simulink library "csu_mpl_mass_properties_lander_lib"  (R2015b)
settings: Solver=ode45  StartTime=0.0  StopTime=10.0  RelTol=1e-3
values from neighbouring files (symbols this model uses):
  mpl_cg_dry = [mpl_cgx_location_fillfrac_0 mpl_cgy_location_fillfrac_0 mpl_cgz_location_fillfrac_0]    [csu_mpl_mass_properties_lander_prep.m]
  mpl_gn2_center_tank1 = [  0.4   0.0   0.2]    [csu_mpl_mass_properties_lander_init.m]
  mpl_gn2_center_tank2 = [  0.0   0.4   0.2]    [csu_mpl_mass_properties_lander_init.m]
  mpl_gn2_center_tank3 = [ -0.4   0.0   0.2]    [csu_mpl_mass_properties_lander_init.m]
  mpl_gn2_center_tank4 = [  0.0  -0.4   0.2]    [csu_mpl_mass_properties_lander_init.m]
  mpl_gn2_cg_table = [ mpl_gn2_cg_fillfrac_0;       mpl_gn2_cg_fillfrac_100   ]    [csu_mpl_mass_properties_lander_prep.m]
  mpl_gn2_drain_efficiency_tank1 = 1.0    (= 1)    [csu_mpl_mass_properties_lander_init.m]
  mpl_gn2_drain_efficiency_tank2 = 1.0    (= 1)    [csu_mpl_mass_properties_lander_init.m]
  mpl_gn2_drain_efficiency_tank3 = 1.0    (= 1)    [csu_mpl_mass_properties_lander_init.m]
  mpl_gn2_drain_efficiency_tank4 = 1.0    (= 1)    [csu_mpl_mass_properties_lander_init.m]
  mpl_gn2_inertia_table_tank1 = [ buildInertiaVector(mpl_gn2_inertia_fillfrac_0_tank1);  buildInertiaVector(mpl_gn2_inertia_fillfrac_100_tank1) ]    [csu_mpl_mass_properties_lander_prep.m]
  mpl_gn2_inertia_table_tank2 = [ buildInertiaVector(mpl_gn2_inertia_fillfrac_0_tank2);  buildInertiaVector(mpl_gn2_inertia_fillfrac_100_tank2) ]    [csu_mpl_mass_properties_lander_prep.m]
  mpl_gn2_inertia_table_tank3 = [ buildInertiaVector(mpl_gn2_inertia_fillfrac_0_tank3);  buildInertiaVector(mpl_gn2_inertia_fillfrac_100_tank3) ]    [csu_mpl_mass_properties_lander_prep.m]
  mpl_gn2_inertia_table_tank4 = [ buildInertiaVector(mpl_gn2_inertia_fillfrac_0_tank4);  buildInertiaVector(mpl_gn2_inertia_fillfrac_100_tank4) ]    [csu_mpl_mass_properties_lander_prep.m]
  mpl_gn2_mass_initial_tank1 = 0.5    [csu_mpl_mass_properties_lander_init.m]    (also in csu_mpl_mass_properties_lander_prep.m = mpl_gn2_mass_initial/4)
  mpl_gn2_mass_initial_tank2 = 0.5    [csu_mpl_mass_properties_lander_init.m]    (also in csu_mpl_mass_properties_lander_prep.m = mpl_gn2_mass_initial/4)
  mpl_gn2_mass_initial_tank3 = 0.5    [csu_mpl_mass_properties_lander_init.m]    (also in csu_mpl_mass_properties_lander_prep.m = mpl_gn2_mass_initial/4)
  mpl_gn2_mass_initial_tank4 = 0.5    [csu_mpl_mass_properties_lander_init.m]    (also in csu_mpl_mass_properties_lander_prep.m = mpl_gn2_mass_initial/4)
  mpl_gn2_mass_table = [ mpl_gn2_mass_fillfrac_0;     mpl_gn2_mass_fillfrac_100 ]    [csu_mpl_mass_properties_lander_prep.m]
  mpl_htp_cg_table = [ mpl_htp_cg_fillfrac_0;     mpl_htp_cg_fillfrac_100   ]    [csu_mpl_mass_properties_lander_prep.m]
  mpl_htp_inertia_table = [ buildInertiaVector(mpl_htp_inertia_fillfrac_0);  buildInertiaVector(mpl_htp_inertia_fillfrac_100) ]    [csu_mpl_mass_properties_lander_prep.m]
  mpl_htp_mass_initial = 317.68    [csu_mpl_mass_properties_lander_init.m]
  mpl_htp_mass_table = [ mpl_htp_mass_fillfrac_0;   mpl_htp_mass_fillfrac_100 ]    [csu_mpl_mass_properties_lander_prep.m]
  mpl_htp_tank_center = [  0.0  0.0  0.4]    [csu_mpl_mass_properties_lander_init.m]
  mpl_inertia_dry = buildInertiaMatrix(mpl_inertia_fillfrac_0([1 2 3 4 6 5]))    [csu_mpl_mass_properties_lander_prep.m]
  mpl_mass_dry = 123.9    [csu_mpl_mass_properties_lander_init_scn_4.m]    (also in csu_mpl_mass_properties_lander_prep.m = mpl_mass_fillfrac_0)
  mpl_rp1_cg_table = [ mpl_rp1_cg_fillfrac_0;     mpl_rp1_cg_fillfrac_100   ]    [csu_mpl_mass_properties_lander_prep.m]
  mpl_rp1_inertia_table = [ buildInertiaVector(mpl_rp1_inertia_fillfrac_0);  buildInertiaVector(mpl_rp1_inertia_fillfrac_100) ]    [csu_mpl_mass_properties_lander_prep.m]
  mpl_rp1_mass_initial = 79.42    [csu_mpl_mass_properties_lander_init.m]
  mpl_rp1_mass_table = [ mpl_rp1_mass_fillfrac_0;   mpl_rp1_mass_fillfrac_100 ]    [csu_mpl_mass_properties_lander_prep.m]
  mpl_rp1_tank_center = [  0.0  0.0  0.1]    [csu_mpl_mass_properties_lander_init.m]
libraries: util_mass_prop_lib x14, simulink x4, util_common_lib x2, util_info_lib x1, util_quat_lib x1
settings Model: Creator=Mark Agbayani  LastModifiedBy=jimkaidy
settings DataIOCC: SaveFormat=Array
settings DebuggingCC: SolverPrmCheckMsg=warning
settings HardwareCC: ProdBitPerPointer=32  ProdLargestAtomicFloat=None  ProdIntDivRoundTo=Undefined  ProdEndianess=Unspecified  ProdWordSize=32  ProdHWDeviceType=32-bit Generic
settings GRTTargetCC: GeneratePreprocessorConditionals=Disable all
settings ConfigComp: CovModelRefEnable=Off  CovSFcnEnable=off

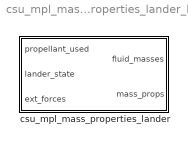
== system csu_mpl_mass_properties_lander_lib ==
  csu_mpl_mass_properties_lander : Subsystem

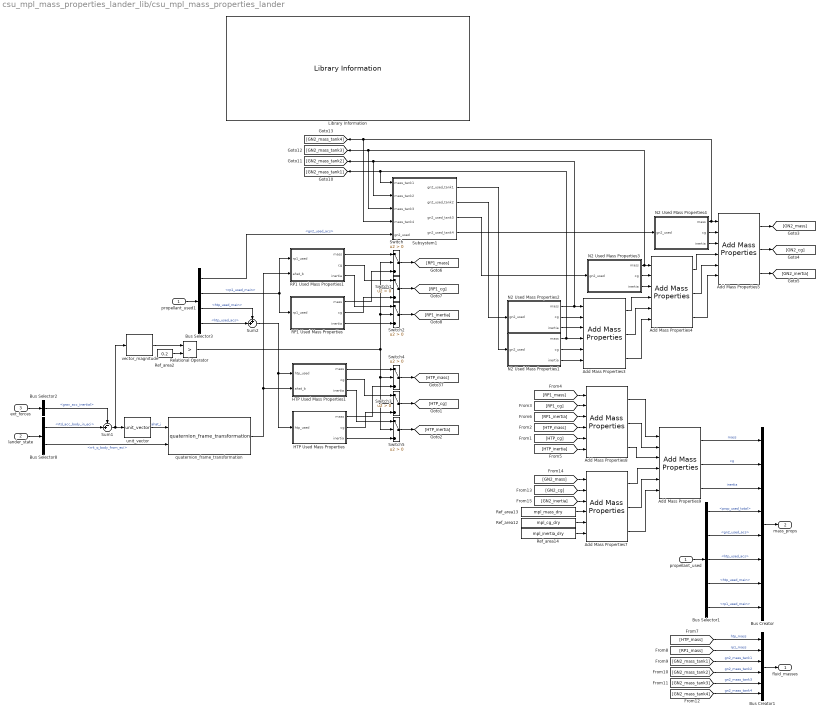
== system csu_mpl_mass_properties_lander_lib/csu_mpl_mass_properties_lander ==
  propellant_used : Inport
  lander_state : Inport  Port=2
  ext_forces : Inport  Port=3
  Add Mass Properties{3..5,7..9} (6 alike) : util_mass_prop_lib/Add Mass Properties  SystemSampleTime=-1
  Bus Creator : BusCreator  Inputs=8  OutDataTypeStr=Bus: mass_props_msg_t
  Bus Creator1 : BusCreator  Inputs=6
  Bus Selector1 : BusSelector  OutputSignals=prop_used_total,gn2_used_acs,htp_used_acs,htp_used_main,rp1_used_main
  Bus Selector2 : BusSelector  OutputSignals=grav_acc_inertial
  Bus Selector3 : BusSelector  OutputSignals=gn2_used_acs,rp1_used_main,htp_used_main,htp_used_acs
  Bus Selector8 : BusSelector  OutputSignals=rtd_acc_body_in_eci,rrk_q_body_from_eci
  HTP Used Mass Properties : Subsystem
  HTP Used Mass Properties1 : Subsystem
  Library Information : util_info_lib/Library Information  owner='NONE'
  N2 Used Mass Properties1 : Subsystem
  N2 Used Mass Properties2 : Subsystem
  N2 Used Mass Properties3 : Subsystem
  N2 Used Mass Properties4 : Subsystem
  RP1 Used Mass Properties : Subsystem
  RP1 Used Mass Properties1 : Subsystem
  Ref_area12 : Constant  Value=mpl_cg_dry
  Ref_area13 : Constant  Value=mpl_mass_dry
  Ref_area14 : Constant  Value=mpl_inertia_dry
  Ref_area2 : Constant  Value=0.2
  Relational Operator : RelationalOperator  Operator=>  OutDataTypeStr=boolean
  Subsystem1 : Subsystem
  Sum1 : Sum  Inputs=-+|
  Sum2 : Sum  Inputs=++|
  Switch{,1..5} (6 alike) : Switch  Criteria=u2 > Threshold
  propellant_used1 : InportShadow
  quaternion_frame_transformation : util_quat_lib/quaternion_frame_transformation  SystemSampleTime=-1
  unit_vector : util_common_lib/unit_vector  SystemSampleTime=-1
  vector_magnitude : util_common_lib/vector_magnitude  SystemSampleTime=-1
  fluid_masses : Outport
  mass_props : Outport  Port=2
  wires:
  Bus Selector8/1 -> Sum1/2  "<rtd_acc_body_in_eci>"
  Bus Selector2/1 -> Sum1/1  "<grav_acc_inertial>"
  ext_forces/1 -> Bus Selector2/1
  Sum1/1 -> unit_vector/1, vector_magnitude/1
  Relational Operator/1 -> Switch2/2, Switch1/2, Switch/2, Switch4/2, Switch5/2, Switch3/2
  Switch3/1 -> [HTP_cg]
  Switch5/1 -> [HTP_inertia]
  Switch4/1 -> [HTP_mass]
  HTP Used Mass Properties/3(inertia) -> Switch5/3
  HTP Used Mass Properties1/3(inertia) -> Switch5/1
  HTP Used Mass Properties/2(cg) -> Switch3/3
  HTP Used Mass Properties1/2(cg) -> Switch3/1
  HTP Used Mass Properties/1(mass) -> Switch4/3
  HTP Used Mass Properties1/1(mass) -> Switch4/1
  RP1 Used Mass Properties/3(inertia) -> Switch2/3
  RP1 Used Mass Properties1/3(inertia) -> Switch2/1
  RP1 Used Mass Properties/2(cg) -> Switch1/3
  RP1 Used Mass Properties1/2(cg) -> Switch1/1
  RP1 Used Mass Properties/1(mass) -> Switch/3
  RP1 Used Mass Properties1/1(mass) -> Switch/1
  Switch2/1 -> [RP1_inertia]
  Switch1/1 -> [RP1_cg]
  Switch/1 -> [RP1_mass]
  Ref_area2/1 -> Relational Operator/2
  vector_magnitude/1 -> Relational Operator/1
  quaternion_frame_transformation/1 -> RP1 Used Mass Properties1/2(ahat_b), HTP Used Mass Properties1/2(ahat_b)
  Bus Selector3/1 -> Subsystem1/5(gn2_used)  "<gn2_used_acs>"
  Bus Selector1/5 -> Bus Creator/8  "<rp1_used_main>"
  Bus Selector1/2 -> Bus Creator/5  "<gn2_used_acs>"
  [GN2_inertia] -> Add Mass Properties7/3
  [GN2_cg] -> Add Mass Properties7/2
  [GN2_mass] -> Add Mass Properties7/1
  Add Mass Properties7/3 -> Add Mass Properties9/6
  Add Mass Properties7/2 -> Add Mass Properties9/5
  Add Mass Properties7/1 -> Add Mass Properties9/4
  Sum2/1 -> HTP Used Mass Properties1/1(htp_used), HTP Used Mass Properties/1(htp_used)
  Bus Selector3/4 -> Sum2/2  "<htp_used_acs>"
  Bus Selector3/2 -> RP1 Used Mass Properties/1(rp1_used), RP1 Used Mass Properties1/1(rp1_used)  "<rp1_used_main>"
  unit_vector/1 -> quaternion_frame_transformation/1  "ahat_i"
  Bus Selector8/2 -> quaternion_frame_transformation/2  "<rrk_q_body_from_eci>"
  lander_state/1 -> Bus Selector8/1
  [GN2_mass_tank4] -> Bus Creator1/6  "gn2_mass_tank4"
  [GN2_mass_tank3] -> Bus Creator1/5  "gn2_mass_tank3"
  [GN2_mass_tank2] -> Bus Creator1/4  "gn2_mass_tank2"
  [GN2_mass_tank1] -> Bus Creator1/3  "gn2_mass_tank1"
  [HTP_mass] -> Bus Creator1/1  "htp_mass"
  Bus Creator1/1 -> fluid_masses/1
  Subsystem1/1(gn2_used_tank1) -> N2 Used Mass Properties1/1(gn2_used)
  Subsystem1/2(gn2_used_tank2) -> N2 Used Mass Properties2/1(gn2_used)
  Subsystem1/3(gn2_used_tank3) -> N2 Used Mass Properties3/1(gn2_used)
  Subsystem1/4(gn2_used_tank4) -> N2 Used Mass Properties4/1(gn2_used)
  Ref_area12/1 -> Add Mass Properties7/5
  N2 Used Mass Properties4/1(mass) -> Add Mass Properties5/1, Subsystem1/4(mass_tank4), [GN2_mass_tank4]
  N2 Used Mass Properties3/1(mass) -> Add Mass Properties4/1, Subsystem1/3(mass_tank3), [GN2_mass_tank3]
  N2 Used Mass Properties2/1(mass) -> Add Mass Properties3/1, Subsystem1/2(mass_tank2), [GN2_mass_tank2]
  N2 Used Mass Properties1/1(mass) -> Add Mass Properties3/4, [GN2_mass_tank1], Subsystem1/1(mass_tank1)
  Ref_area13/1 -> Add Mass Properties7/4
  Ref_area14/1 -> Add Mass Properties7/6
  N2 Used Mass Properties1/2(cg) -> Add Mass Properties3/5
  N2 Used Mass Properties1/3(inertia) -> Add Mass Properties3/6
  N2 Used Mass Properties2/3(inertia) -> Add Mass Properties3/3
  N2 Used Mass Properties2/2(cg) -> Add Mass Properties3/2
  Add Mass Properties3/1 -> Add Mass Properties4/4
  Add Mass Properties3/2 -> Add Mass Properties4/5
  Add Mass Properties3/3 -> Add Mass Properties4/6
  N2 Used Mass Properties3/3(inertia) -> Add Mass Properties4/3
  N2 Used Mass Properties3/2(cg) -> Add Mass Properties4/2
  N2 Used Mass Properties4/2(cg) -> Add Mass Properties5/2
  N2 Used Mass Properties4/3(inertia) -> Add Mass Properties5/3
  Add Mass Properties4/1 -> Add Mass Properties5/4
  Add Mass Properties4/2 -> Add Mass Properties5/5
  Add Mass Properties4/3 -> Add Mass Properties5/6
  Add Mass Properties5/1 -> [GN2_mass]
  Add Mass Properties5/2 -> [GN2_cg]
  Add Mass Properties5/3 -> [GN2_inertia]
  [HTP_inertia] -> Add Mass Properties8/6
  [HTP_cg] -> Add Mass Properties8/5
  [HTP_mass] -> Add Mass Properties8/4
  [RP1_inertia] -> Add Mass Properties8/3
  [RP1_cg] -> Add Mass Properties8/2
  [RP1_mass] -> Add Mass Properties8/1
  Add Mass Properties8/3 -> Add Mass Properties9/3
  Add Mass Properties8/2 -> Add Mass Properties9/2
  Add Mass Properties8/1 -> Add Mass Properties9/1
  Bus Selector3/3 -> Sum2/1  "<htp_used_main>"
  Bus Creator/1 -> mass_props/1
  Bus Selector1/1 -> Bus Creator/4  "<prop_used_total>"
  Bus Selector1/3 -> Bus Creator/6  "<htp_used_acs>"
  Bus Selector1/4 -> Bus Creator/7  "<htp_used_main>"
  Add Mass Properties9/1 -> Bus Creator/1  "mass"
  Add Mass Properties9/2 -> Bus Creator/2  "cg"
  Add Mass Properties9/3 -> Bus Creator/3  "inertia"
  propellant_used/1 -> Bus Selector1/1
  propellant_used1/1 -> Bus Selector3/1
  [RP1_mass] -> Bus Creator1/2  "rp1_mass"

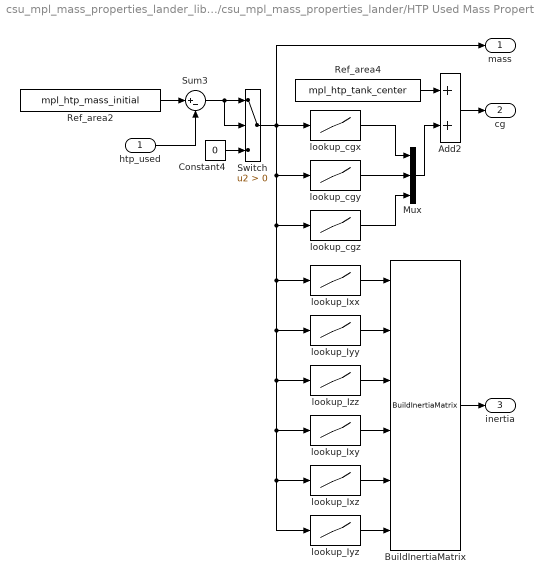
== system csu_mpl_mass_properties_lander_lib/csu_mpl_mass_properties_lander/HTP Used Mass Properties ==
  htp_used : Inport
  Add2 : Sum
  BuildInertiaMatrix : util_mass_prop_lib/BuildInertiaMatrix  SystemSampleTime=-1
  Constant4 : Constant  Value=0
  Mux : Mux  Inputs=3
  Ref_area2 : Constant  Value=mpl_htp_mass_initial
  Ref_area4 : Constant  Value=mpl_htp_tank_center
  Sum3 : Sum  Inputs=|+-
  Switch : Switch  Criteria=u2 > Threshold  SaturateOnIntegerOverflow=on
  lookup_Ixx : Lookup  InputValues=mpl_htp_mass_table  Table=mpl_htp_inertia_table(:,1)
  lookup_Ixy : Lookup  InputValues=mpl_htp_mass_table  Table=mpl_htp_inertia_table(:,4)
  lookup_Ixz : Lookup  InputValues=mpl_htp_mass_table  Table=mpl_htp_inertia_table(:,5)
  lookup_Iyy : Lookup  InputValues=mpl_htp_mass_table  Table=mpl_htp_inertia_table(:,2)
  lookup_Iyz : Lookup  InputValues=mpl_htp_mass_table  Table=mpl_htp_inertia_table(:,6)
  lookup_Izz : Lookup  InputValues=mpl_htp_mass_table  Table=mpl_htp_inertia_table(:,3)
  lookup_cgx : Lookup  InputValues=mpl_htp_mass_table  Table=mpl_htp_cg_table(:,1)
  lookup_cgy : Lookup  InputValues=mpl_htp_mass_table  Table=mpl_htp_cg_table(:,2)
  lookup_cgz : Lookup  InputValues=mpl_htp_mass_table  Table=mpl_htp_cg_table(:,3)
  mass : Outport
  cg : Outport  Port=2
  inertia : Outport  Port=3
  wires:
  Mux/1 -> Add2/2
  lookup_cgy/1 -> Mux/2
  lookup_cgz/1 -> Mux/3
  Ref_area4/1 -> Add2/1
  lookup_Ixx/1 -> BuildInertiaMatrix/1
  lookup_Iyy/1 -> BuildInertiaMatrix/2
  lookup_Izz/1 -> BuildInertiaMatrix/3
  lookup_Ixy/1 -> BuildInertiaMatrix/4
  lookup_Ixz/1 -> BuildInertiaMatrix/5
  lookup_Iyz/1 -> BuildInertiaMatrix/6
  BuildInertiaMatrix/1 -> inertia/1
  lookup_cgx/1 -> Mux/1
  Ref_area2/1 -> Sum3/1
  htp_used/1 -> Sum3/2
  Add2/1 -> cg/1
  Switch/1 -> mass/1, lookup_cgx/1, lookup_cgy/1, lookup_cgz/1, lookup_Ixx/1, lookup_Iyy/1, lookup_Izz/1, lookup_Ixy/1, lookup_Ixz/1, lookup_Iyz/1
  Sum3/1 -> Switch/2, Switch/1
  Constant4/1 -> Switch/3

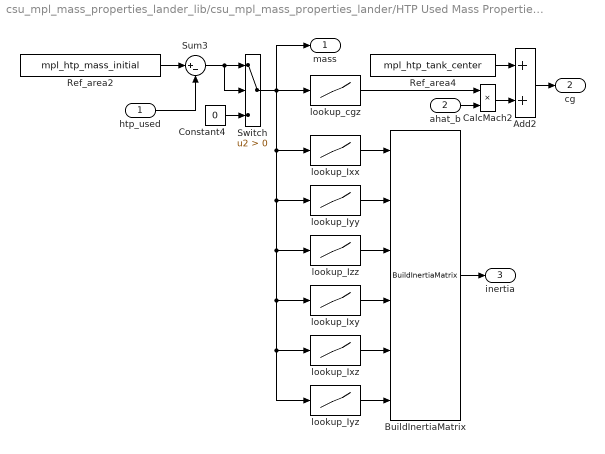
== system csu_mpl_mass_properties_lander_lib/csu_mpl_mass_properties_lander/HTP Used Mass Properties1 ==
  htp_used : Inport
  ahat_b : Inport  Port=2
  Add2 : Sum
  BuildInertiaMatrix : util_mass_prop_lib/BuildInertiaMatrix  SystemSampleTime=-1
  CalcMach2 : Product  SaturateOnIntegerOverflow=on  OutDataTypeStr=Inherit: Same as first input
  Constant4 : Constant  Value=0
  Ref_area2 : Constant  Value=mpl_htp_mass_initial
  Ref_area4 : Constant  Value=mpl_htp_tank_center
  Sum3 : Sum  Inputs=|+-
  Switch : Switch  Criteria=u2 > Threshold  SaturateOnIntegerOverflow=on
  lookup_Ixx : Lookup  InputValues=mpl_htp_mass_table  Table=mpl_htp_inertia_table(:,1)
  lookup_Ixy : Lookup  InputValues=mpl_htp_mass_table  Table=mpl_htp_inertia_table(:,4)
  lookup_Ixz : Lookup  InputValues=mpl_htp_mass_table  Table=mpl_htp_inertia_table(:,5)
  lookup_Iyy : Lookup  InputValues=mpl_htp_mass_table  Table=mpl_htp_inertia_table(:,2)
  lookup_Iyz : Lookup  InputValues=mpl_htp_mass_table  Table=mpl_htp_inertia_table(:,6)
  lookup_Izz : Lookup  InputValues=mpl_htp_mass_table  Table=mpl_htp_inertia_table(:,3)
  lookup_cgz : Lookup  InputValues=mpl_htp_mass_table  Table=mpl_htp_cg_table(:,3)
  mass : Outport
  cg : Outport  Port=2
  inertia : Outport  Port=3
  wires:
  Add2/1 -> cg/1
  htp_used/1 -> Sum3/2
  Ref_area2/1 -> Sum3/1
  BuildInertiaMatrix/1 -> inertia/1
  lookup_Iyz/1 -> BuildInertiaMatrix/6
  lookup_Ixz/1 -> BuildInertiaMatrix/5
  lookup_Ixy/1 -> BuildInertiaMatrix/4
  lookup_Izz/1 -> BuildInertiaMatrix/3
  lookup_Iyy/1 -> BuildInertiaMatrix/2
  lookup_Ixx/1 -> BuildInertiaMatrix/1
  Ref_area4/1 -> Add2/1
  CalcMach2/1 -> Add2/2
  Switch/1 -> mass/1, lookup_Iyz/1, lookup_Ixz/1, lookup_Ixy/1, lookup_Izz/1, lookup_Iyy/1, lookup_Ixx/1, lookup_cgz/1
  Sum3/1 -> Switch/2, Switch/1
  Constant4/1 -> Switch/3
  lookup_cgz/1 -> CalcMach2/1
  ahat_b/1 -> CalcMach2/2

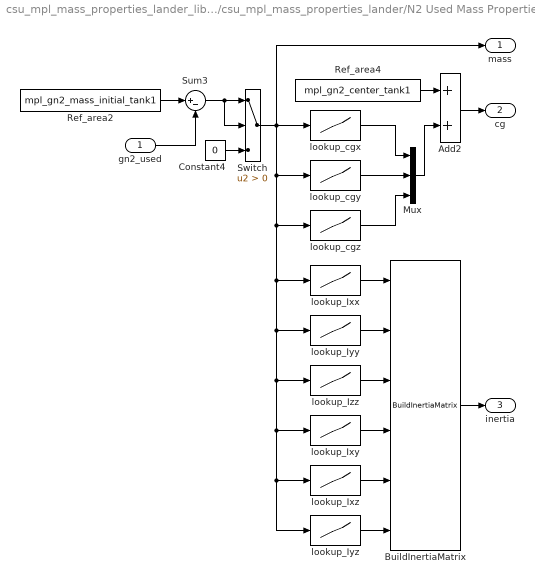
== system csu_mpl_mass_properties_lander_lib/csu_mpl_mass_properties_lander/N2 Used Mass Properties1 ==
  gn2_used : Inport
  Add2 : Sum
  BuildInertiaMatrix : util_mass_prop_lib/BuildInertiaMatrix  SystemSampleTime=-1
  Constant4 : Constant  Value=0
  Mux : Mux  Inputs=3
  Ref_area2 : Constant  Value=mpl_gn2_mass_initial_tank1
  Ref_area4 : Constant  Value=mpl_gn2_center_tank1
  Sum3 : Sum  Inputs=|+-
  Switch : Switch  Criteria=u2 > Threshold  SaturateOnIntegerOverflow=on
  lookup_Ixx : Lookup  InputValues=mpl_gn2_mass_table  Table=mpl_gn2_inertia_table_tank1(:,1)
  lookup_Ixy : Lookup  InputValues=mpl_gn2_mass_table  Table=mpl_gn2_inertia_table_tank1(:,4)
  lookup_Ixz : Lookup  InputValues=mpl_gn2_mass_table  Table=mpl_gn2_inertia_table_tank1(:,5)
  lookup_Iyy : Lookup  InputValues=mpl_gn2_mass_table  Table=mpl_gn2_inertia_table_tank1(:,2)
  lookup_Iyz : Lookup  InputValues=mpl_gn2_mass_table  Table=mpl_gn2_inertia_table_tank1(:,6)
  lookup_Izz : Lookup  InputValues=mpl_gn2_mass_table  Table=mpl_gn2_inertia_table_tank1(:,3)
  lookup_cgx : Lookup  InputValues=mpl_gn2_mass_table  Table=mpl_gn2_cg_table(:,1)
  lookup_cgy : Lookup  InputValues=mpl_gn2_mass_table  Table=mpl_gn2_cg_table(:,2)
  lookup_cgz : Lookup  InputValues=mpl_gn2_mass_table  Table=mpl_gn2_cg_table(:,3)
  mass : Outport
  cg : Outport  Port=2
  inertia : Outport  Port=3
  wires:
  Constant4/1 -> Switch/3
  Sum3/1 -> Switch/1, Switch/2
  Switch/1 -> lookup_Iyz/1, lookup_Ixz/1, lookup_Ixy/1, lookup_Izz/1, lookup_Iyy/1, lookup_Ixx/1, lookup_cgz/1, lookup_cgy/1, lookup_cgx/1, mass/1
  Add2/1 -> cg/1
  gn2_used/1 -> Sum3/2
  Ref_area2/1 -> Sum3/1
  lookup_cgx/1 -> Mux/1
  BuildInertiaMatrix/1 -> inertia/1
  lookup_Iyz/1 -> BuildInertiaMatrix/6
  lookup_Ixz/1 -> BuildInertiaMatrix/5
  lookup_Ixy/1 -> BuildInertiaMatrix/4
  lookup_Izz/1 -> BuildInertiaMatrix/3
  lookup_Iyy/1 -> BuildInertiaMatrix/2
  lookup_Ixx/1 -> BuildInertiaMatrix/1
  Ref_area4/1 -> Add2/1
  lookup_cgz/1 -> Mux/3
  lookup_cgy/1 -> Mux/2
  Mux/1 -> Add2/2

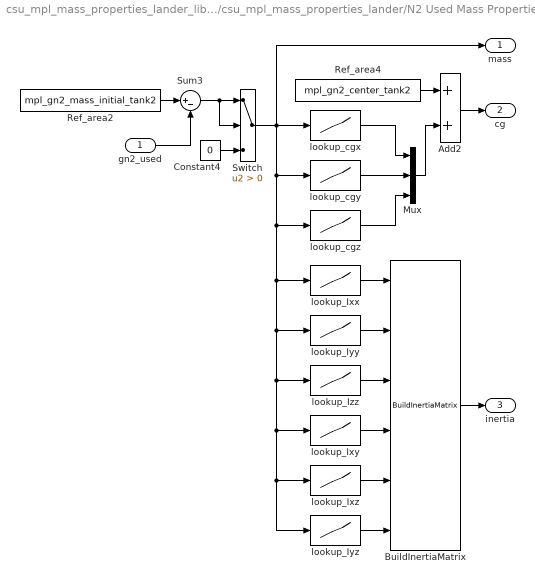
== system csu_mpl_mass_properties_lander_lib/csu_mpl_mass_properties_lander/N2 Used Mass Properties2 ==
  gn2_used : Inport
  Add2 : Sum
  BuildInertiaMatrix : util_mass_prop_lib/BuildInertiaMatrix  SystemSampleTime=-1
  Constant4 : Constant  Value=0
  Mux : Mux  Inputs=3
  Ref_area2 : Constant  Value=mpl_gn2_mass_initial_tank2
  Ref_area4 : Constant  Value=mpl_gn2_center_tank2
  Sum3 : Sum  Inputs=|+-
  Switch : Switch  Criteria=u2 > Threshold  SaturateOnIntegerOverflow=on
  lookup_Ixx : Lookup  InputValues=mpl_gn2_mass_table  Table=mpl_gn2_inertia_table_tank2(:,1)
  lookup_Ixy : Lookup  InputValues=mpl_gn2_mass_table  Table=mpl_gn2_inertia_table_tank2(:,4)
  lookup_Ixz : Lookup  InputValues=mpl_gn2_mass_table  Table=mpl_gn2_inertia_table_tank2(:,5)
  lookup_Iyy : Lookup  InputValues=mpl_gn2_mass_table  Table=mpl_gn2_inertia_table_tank2(:,2)
  lookup_Iyz : Lookup  InputValues=mpl_gn2_mass_table  Table=mpl_gn2_inertia_table_tank2(:,6)
  lookup_Izz : Lookup  InputValues=mpl_gn2_mass_table  Table=mpl_gn2_inertia_table_tank2(:,3)
  lookup_cgx : Lookup  InputValues=mpl_gn2_mass_table  Table=mpl_gn2_cg_table(:,1)
  lookup_cgy : Lookup  InputValues=mpl_gn2_mass_table  Table=mpl_gn2_cg_table(:,2)
  lookup_cgz : Lookup  InputValues=mpl_gn2_mass_table  Table=mpl_gn2_cg_table(:,3)
  mass : Outport
  cg : Outport  Port=2
  inertia : Outport  Port=3
  wires:
  Constant4/1 -> Switch/3
  Sum3/1 -> Switch/1, Switch/2
  Switch/1 -> lookup_cgx/1, lookup_cgy/1, lookup_cgz/1, lookup_Ixx/1, lookup_Iyy/1, lookup_Izz/1, lookup_Ixy/1, lookup_Ixz/1, lookup_Iyz/1, mass/1
  Mux/1 -> Add2/2
  lookup_cgy/1 -> Mux/2
  lookup_cgz/1 -> Mux/3
  Ref_area4/1 -> Add2/1
  lookup_Ixx/1 -> BuildInertiaMatrix/1
  lookup_Iyy/1 -> BuildInertiaMatrix/2
  lookup_Izz/1 -> BuildInertiaMatrix/3
  lookup_Ixy/1 -> BuildInertiaMatrix/4
  lookup_Ixz/1 -> BuildInertiaMatrix/5
  lookup_Iyz/1 -> BuildInertiaMatrix/6
  BuildInertiaMatrix/1 -> inertia/1
  lookup_cgx/1 -> Mux/1
  Ref_area2/1 -> Sum3/1
  gn2_used/1 -> Sum3/2
  Add2/1 -> cg/1

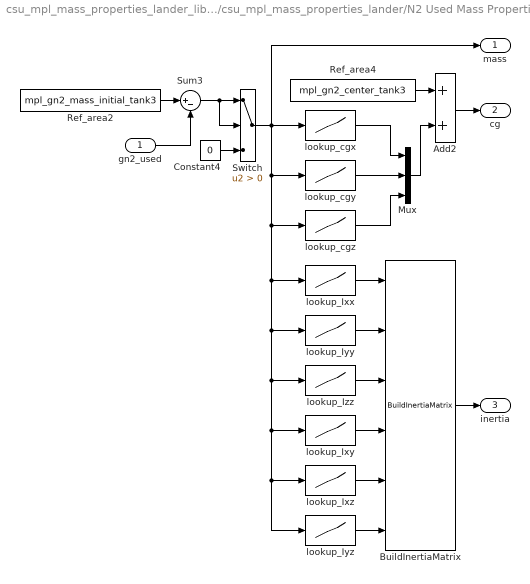
== system csu_mpl_mass_properties_lander_lib/csu_mpl_mass_properties_lander/N2 Used Mass Properties3 ==
  gn2_used : Inport
  Add2 : Sum
  BuildInertiaMatrix : util_mass_prop_lib/BuildInertiaMatrix  SystemSampleTime=-1
  Constant4 : Constant  Value=0
  Mux : Mux  Inputs=3
  Ref_area2 : Constant  Value=mpl_gn2_mass_initial_tank3
  Ref_area4 : Constant  Value=mpl_gn2_center_tank3
  Sum3 : Sum  Inputs=|+-
  Switch : Switch  Criteria=u2 > Threshold  SaturateOnIntegerOverflow=on
  lookup_Ixx : Lookup  InputValues=mpl_gn2_mass_table  Table=mpl_gn2_inertia_table_tank3(:,1)
  lookup_Ixy : Lookup  InputValues=mpl_gn2_mass_table  Table=mpl_gn2_inertia_table_tank3(:,4)
  lookup_Ixz : Lookup  InputValues=mpl_gn2_mass_table  Table=mpl_gn2_inertia_table_tank3(:,5)
  lookup_Iyy : Lookup  InputValues=mpl_gn2_mass_table  Table=mpl_gn2_inertia_table_tank3(:,2)
  lookup_Iyz : Lookup  InputValues=mpl_gn2_mass_table  Table=mpl_gn2_inertia_table_tank3(:,6)
  lookup_Izz : Lookup  InputValues=mpl_gn2_mass_table  Table=mpl_gn2_inertia_table_tank3(:,3)
  lookup_cgx : Lookup  InputValues=mpl_gn2_mass_table  Table=mpl_gn2_cg_table(:,1)
  lookup_cgy : Lookup  InputValues=mpl_gn2_mass_table  Table=mpl_gn2_cg_table(:,2)
  lookup_cgz : Lookup  InputValues=mpl_gn2_mass_table  Table=mpl_gn2_cg_table(:,3)
  mass : Outport
  cg : Outport  Port=2
  inertia : Outport  Port=3
  wires:
  Constant4/1 -> Switch/3
  Sum3/1 -> Switch/1, Switch/2
  Switch/1 -> lookup_cgx/1, mass/1, lookup_Iyz/1, lookup_Ixz/1, lookup_Ixy/1, lookup_Izz/1, lookup_Iyy/1, lookup_Ixx/1, lookup_cgz/1, lookup_cgy/1
  Add2/1 -> cg/1
  gn2_used/1 -> Sum3/2
  Ref_area2/1 -> Sum3/1
  lookup_cgx/1 -> Mux/1
  BuildInertiaMatrix/1 -> inertia/1
  lookup_Iyz/1 -> BuildInertiaMatrix/6
  lookup_Ixz/1 -> BuildInertiaMatrix/5
  lookup_Ixy/1 -> BuildInertiaMatrix/4
  lookup_Izz/1 -> BuildInertiaMatrix/3
  lookup_Iyy/1 -> BuildInertiaMatrix/2
  lookup_Ixx/1 -> BuildInertiaMatrix/1
  Ref_area4/1 -> Add2/1
  lookup_cgz/1 -> Mux/3
  lookup_cgy/1 -> Mux/2
  Mux/1 -> Add2/2

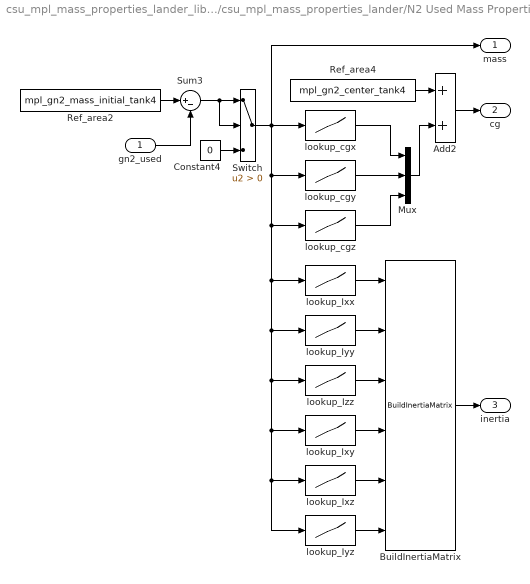
== system csu_mpl_mass_properties_lander_lib/csu_mpl_mass_properties_lander/N2 Used Mass Properties4 ==
  gn2_used : Inport
  Add2 : Sum
  BuildInertiaMatrix : util_mass_prop_lib/BuildInertiaMatrix  SystemSampleTime=-1
  Constant4 : Constant  Value=0
  Mux : Mux  Inputs=3
  Ref_area2 : Constant  Value=mpl_gn2_mass_initial_tank4
  Ref_area4 : Constant  Value=mpl_gn2_center_tank4
  Sum3 : Sum  Inputs=|+-
  Switch : Switch  Criteria=u2 > Threshold  SaturateOnIntegerOverflow=on
  lookup_Ixx : Lookup  InputValues=mpl_gn2_mass_table  Table=mpl_gn2_inertia_table_tank4(:,1)
  lookup_Ixy : Lookup  InputValues=mpl_gn2_mass_table  Table=mpl_gn2_inertia_table_tank4(:,4)
  lookup_Ixz : Lookup  InputValues=mpl_gn2_mass_table  Table=mpl_gn2_inertia_table_tank4(:,5)
  lookup_Iyy : Lookup  InputValues=mpl_gn2_mass_table  Table=mpl_gn2_inertia_table_tank4(:,2)
  lookup_Iyz : Lookup  InputValues=mpl_gn2_mass_table  Table=mpl_gn2_inertia_table_tank4(:,6)
  lookup_Izz : Lookup  InputValues=mpl_gn2_mass_table  Table=mpl_gn2_inertia_table_tank4(:,3)
  lookup_cgx : Lookup  InputValues=mpl_gn2_mass_table  Table=mpl_gn2_cg_table(:,1)
  lookup_cgy : Lookup  InputValues=mpl_gn2_mass_table  Table=mpl_gn2_cg_table(:,2)
  lookup_cgz : Lookup  InputValues=mpl_gn2_mass_table  Table=mpl_gn2_cg_table(:,3)
  mass : Outport
  cg : Outport  Port=2
  inertia : Outport  Port=3
  wires:
  Constant4/1 -> Switch/3
  Sum3/1 -> Switch/1, Switch/2
  Switch/1 -> lookup_cgx/1, mass/1, lookup_cgy/1, lookup_cgz/1, lookup_Ixx/1, lookup_Iyy/1, lookup_Izz/1, lookup_Ixy/1, lookup_Ixz/1, lookup_Iyz/1
  Mux/1 -> Add2/2
  lookup_cgy/1 -> Mux/2
  lookup_cgz/1 -> Mux/3
  Ref_area4/1 -> Add2/1
  lookup_Ixx/1 -> BuildInertiaMatrix/1
  lookup_Iyy/1 -> BuildInertiaMatrix/2
  lookup_Izz/1 -> BuildInertiaMatrix/3
  lookup_Ixy/1 -> BuildInertiaMatrix/4
  lookup_Ixz/1 -> BuildInertiaMatrix/5
  lookup_Iyz/1 -> BuildInertiaMatrix/6
  BuildInertiaMatrix/1 -> inertia/1
  lookup_cgx/1 -> Mux/1
  Ref_area2/1 -> Sum3/1
  gn2_used/1 -> Sum3/2
  Add2/1 -> cg/1

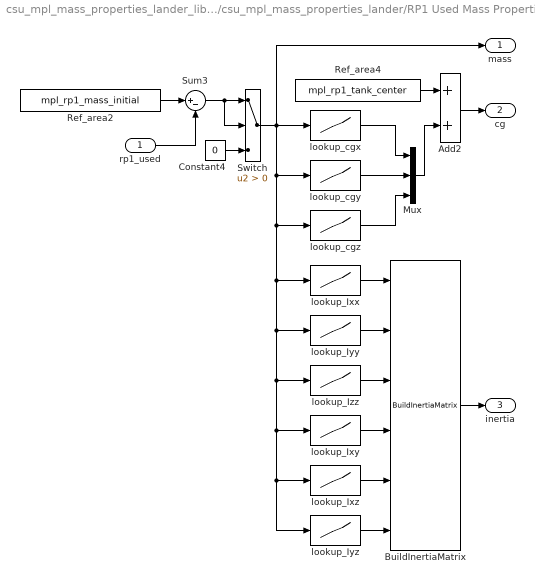
== system csu_mpl_mass_properties_lander_lib/csu_mpl_mass_properties_lander/RP1 Used Mass Properties ==
  rp1_used : Inport
  Add2 : Sum
  BuildInertiaMatrix : util_mass_prop_lib/BuildInertiaMatrix  SystemSampleTime=-1
  Constant4 : Constant  Value=0
  Mux : Mux  Inputs=3
  Ref_area2 : Constant  Value=mpl_rp1_mass_initial
  Ref_area4 : Constant  Value=mpl_rp1_tank_center
  Sum3 : Sum  Inputs=|+-
  Switch : Switch  Criteria=u2 > Threshold  SaturateOnIntegerOverflow=on
  lookup_Ixx : Lookup  InputValues=mpl_rp1_mass_table  Table=mpl_rp1_inertia_table(:,1)
  lookup_Ixy : Lookup  InputValues=mpl_rp1_mass_table  Table=mpl_rp1_inertia_table(:,4)
  lookup_Ixz : Lookup  InputValues=mpl_rp1_mass_table  Table=mpl_rp1_inertia_table(:,5)
  lookup_Iyy : Lookup  InputValues=mpl_rp1_mass_table  Table=mpl_rp1_inertia_table(:,2)
  lookup_Iyz : Lookup  InputValues=mpl_rp1_mass_table  Table=mpl_rp1_inertia_table(:,6)
  lookup_Izz : Lookup  InputValues=mpl_rp1_mass_table  Table=mpl_rp1_inertia_table(:,3)
  lookup_cgx : Lookup  InputValues=mpl_rp1_mass_table  Table=mpl_rp1_cg_table(:,1)
  lookup_cgy : Lookup  InputValues=mpl_rp1_mass_table  Table=mpl_rp1_cg_table(:,2)
  lookup_cgz : Lookup  InputValues=mpl_rp1_mass_table  Table=mpl_rp1_cg_table(:,3)
  mass : Outport
  cg : Outport  Port=2
  inertia : Outport  Port=3
  wires:
  Constant4/1 -> Switch/3
  Sum3/1 -> Switch/1, Switch/2
  Switch/1 -> lookup_Iyz/1, lookup_Ixz/1, lookup_Ixy/1, lookup_Izz/1, lookup_Iyy/1, lookup_Ixx/1, lookup_cgz/1, lookup_cgy/1, lookup_cgx/1, mass/1
  Add2/1 -> cg/1
  rp1_used/1 -> Sum3/2
  Ref_area2/1 -> Sum3/1
  lookup_cgx/1 -> Mux/1
  BuildInertiaMatrix/1 -> inertia/1
  lookup_Iyz/1 -> BuildInertiaMatrix/6
  lookup_Ixz/1 -> BuildInertiaMatrix/5
  lookup_Ixy/1 -> BuildInertiaMatrix/4
  lookup_Izz/1 -> BuildInertiaMatrix/3
  lookup_Iyy/1 -> BuildInertiaMatrix/2
  lookup_Ixx/1 -> BuildInertiaMatrix/1
  Ref_area4/1 -> Add2/1
  lookup_cgz/1 -> Mux/3
  lookup_cgy/1 -> Mux/2
  Mux/1 -> Add2/2

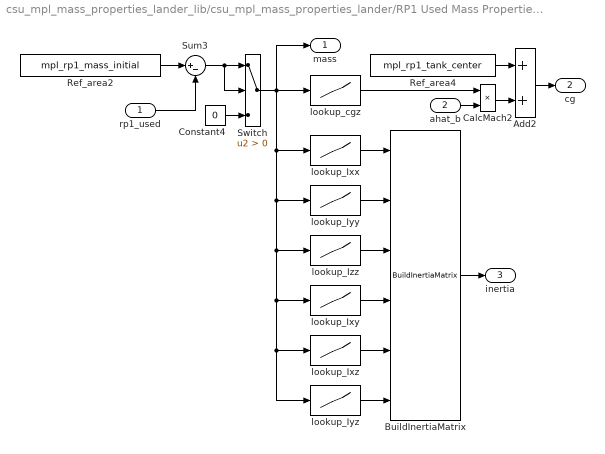
== system csu_mpl_mass_properties_lander_lib/csu_mpl_mass_properties_lander/RP1 Used Mass Properties1 ==
  rp1_used : Inport
  ahat_b : Inport  Port=2
  Add2 : Sum
  BuildInertiaMatrix : util_mass_prop_lib/BuildInertiaMatrix  SystemSampleTime=-1
  CalcMach2 : Product  SaturateOnIntegerOverflow=on  OutDataTypeStr=Inherit: Same as first input
  Constant4 : Constant  Value=0
  Ref_area2 : Constant  Value=mpl_rp1_mass_initial
  Ref_area4 : Constant  Value=mpl_rp1_tank_center
  Sum3 : Sum  Inputs=|+-
  Switch : Switch  Criteria=u2 > Threshold  SaturateOnIntegerOverflow=on
  lookup_Ixx : Lookup  InputValues=mpl_rp1_mass_table  Table=mpl_rp1_inertia_table(:,1)
  lookup_Ixy : Lookup  InputValues=mpl_rp1_mass_table  Table=mpl_rp1_inertia_table(:,4)
  lookup_Ixz : Lookup  InputValues=mpl_rp1_mass_table  Table=mpl_rp1_inertia_table(:,5)
  lookup_Iyy : Lookup  InputValues=mpl_rp1_mass_table  Table=mpl_rp1_inertia_table(:,2)
  lookup_Iyz : Lookup  InputValues=mpl_rp1_mass_table  Table=mpl_rp1_inertia_table(:,6)
  lookup_Izz : Lookup  InputValues=mpl_rp1_mass_table  Table=mpl_rp1_inertia_table(:,3)
  lookup_cgz : Lookup  InputValues=mpl_rp1_mass_table  Table=mpl_rp1_cg_table(:,3)
  mass : Outport
  cg : Outport  Port=2
  inertia : Outport  Port=3
  wires:
  ahat_b/1 -> CalcMach2/2
  lookup_cgz/1 -> CalcMach2/1
  Constant4/1 -> Switch/3
  Sum3/1 -> Switch/1, Switch/2
  Switch/1 -> lookup_cgz/1, lookup_Ixx/1, lookup_Iyy/1, lookup_Izz/1, lookup_Ixy/1, lookup_Ixz/1, lookup_Iyz/1, mass/1
  CalcMach2/1 -> Add2/2
  Ref_area4/1 -> Add2/1
  lookup_Ixx/1 -> BuildInertiaMatrix/1
  lookup_Iyy/1 -> BuildInertiaMatrix/2
  lookup_Izz/1 -> BuildInertiaMatrix/3
  lookup_Ixy/1 -> BuildInertiaMatrix/4
  lookup_Ixz/1 -> BuildInertiaMatrix/5
  lookup_Iyz/1 -> BuildInertiaMatrix/6
  BuildInertiaMatrix/1 -> inertia/1
  Ref_area2/1 -> Sum3/1
  rp1_used/1 -> Sum3/2
  Add2/1 -> cg/1

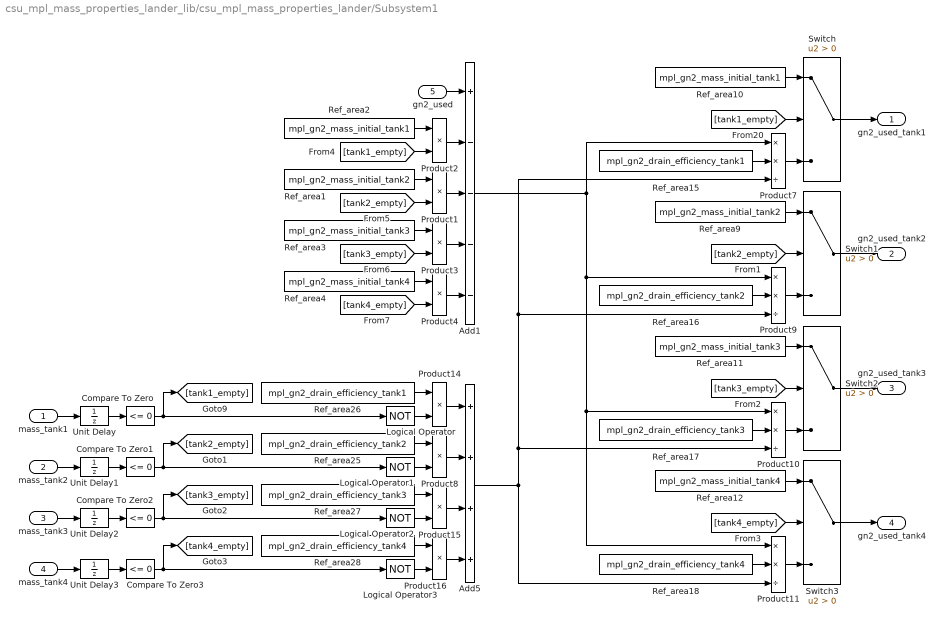
== system csu_mpl_mass_properties_lander_lib/csu_mpl_mass_properties_lander/Subsystem1 ==
  mass_tank1 : Inport
  mass_tank2 : Inport  Port=2
  mass_tank3 : Inport  Port=3
  mass_tank4 : Inport  Port=4
  gn2_used : Inport  Port=5
  Add1 : Sum  Inputs=+----
  Add5 : Sum  Inputs=++++  AccumDataTypeStr=double  OutDataTypeStr=double
  Compare To Zero{,1..3} (4 alike) : simulink/Logic and Bit Operations/Compare To Zero  relop=<=  OutDataTypeStr=boolean
  Logical Operator{,1..3} (4 alike) : Logic  Operator=NOT  AllPortsSameDT=off  OutDataTypeStr=boolean
  Product{1..4,8,14..16} (8 alike) : Product  OutDataTypeStr=double  RndMeth=Zero
  Product{7,9..11} (4 alike) : Product  Inputs=**/  OutDataTypeStr=double  RndMeth=Zero
  Ref_area1 : Constant  Value=mpl_gn2_mass_initial_tank2  OutDataTypeStr=double
  Ref_area10 : Constant  Value=mpl_gn2_mass_initial_tank1  OutDataTypeStr=double
  Ref_area11 : Constant  Value=mpl_gn2_mass_initial_tank3  OutDataTypeStr=double
  Ref_area12 : Constant  Value=mpl_gn2_mass_initial_tank4  OutDataTypeStr=double
  Ref_area15 : Constant  Value=mpl_gn2_drain_efficiency_tank1  OutDataTypeStr=double
  Ref_area16 : Constant  Value=mpl_gn2_drain_efficiency_tank2  OutDataTypeStr=double
  Ref_area17 : Constant  Value=mpl_gn2_drain_efficiency_tank3  OutDataTypeStr=double
  Ref_area18 : Constant  Value=mpl_gn2_drain_efficiency_tank4  OutDataTypeStr=double
  Ref_area2 : Constant  Value=mpl_gn2_mass_initial_tank1  OutDataTypeStr=double
  Ref_area25 : Constant  Value=mpl_gn2_drain_efficiency_tank2  OutDataTypeStr=double
  Ref_area26 : Constant  Value=mpl_gn2_drain_efficiency_tank1  OutDataTypeStr=double
  Ref_area27 : Constant  Value=mpl_gn2_drain_efficiency_tank3  OutDataTypeStr=double
  Ref_area28 : Constant  Value=mpl_gn2_drain_efficiency_tank4  OutDataTypeStr=double
  Ref_area3 : Constant  Value=mpl_gn2_mass_initial_tank3  OutDataTypeStr=double
  Ref_area4 : Constant  Value=mpl_gn2_mass_initial_tank4  OutDataTypeStr=double
  Ref_area9 : Constant  Value=mpl_gn2_mass_initial_tank2  OutDataTypeStr=double
  Switch{,1..3} (4 alike) : Switch  Criteria=u2 > Threshold
  Unit Delay : UnitDelay  InitialCondition=mpl_gn2_mass_initial_tank1  SampleTime=-1
  Unit Delay1 : UnitDelay  InitialCondition=mpl_gn2_mass_initial_tank2  SampleTime=-1
  Unit Delay2 : UnitDelay  InitialCondition=mpl_gn2_mass_initial_tank3  SampleTime=-1
  Unit Delay3 : UnitDelay  InitialCondition=mpl_gn2_mass_initial_tank4  SampleTime=-1
  gn2_used_tank1 : Outport
  gn2_used_tank2 : Outport  Port=2
  gn2_used_tank3 : Outport  Port=3
  gn2_used_tank4 : Outport  Port=4
  wires:
  Unit Delay3/1 -> Compare To Zero3/1
  Unit Delay2/1 -> Compare To Zero2/1
  Unit Delay1/1 -> Compare To Zero1/1
  Unit Delay/1 -> Compare To Zero/1
  Compare To Zero/1 -> [tank1_empty], Logical Operator/1
  Compare To Zero3/1 -> [tank4_empty], Logical Operator3/1
  Compare To Zero2/1 -> [tank3_empty], Logical Operator2/1
  Compare To Zero1/1 -> [tank2_empty], Logical Operator1/1
  [tank4_empty] -> Product4/2
  [tank3_empty] -> Product3/2
  [tank2_empty] -> Product1/2
  [tank1_empty] -> Product2/2
  Ref_area4/1 -> Product4/1
  Ref_area3/1 -> Product3/1
  Ref_area1/1 -> Product1/1
  Product1/1 -> Add1/3
  Product3/1 -> Add1/4
  Product4/1 -> Add1/5
  Product2/1 -> Add1/2
  Ref_area2/1 -> Product2/1
  gn2_used/1 -> Add1/1
  mass_tank4/1 -> Unit Delay3/1
  mass_tank3/1 -> Unit Delay2/1
  mass_tank2/1 -> Unit Delay1/1
  mass_tank1/1 -> Unit Delay/1
  Ref_area28/1 -> Product16/1
  Ref_area27/1 -> Product15/1
  Ref_area25/1 -> Product8/1
  Ref_area26/1 -> Product14/1
  Product16/1 -> Add5/4
  Product15/1 -> Add5/3
  Product8/1 -> Add5/2
  Product14/1 -> Add5/1
  Logical Operator/1 -> Product14/2
  Logical Operator1/1 -> Product8/2
  Logical Operator2/1 -> Product15/2
  Logical Operator3/1 -> Product16/2
  Ref_area12/1 -> Switch3/1
  [tank4_empty] -> Switch3/2
  Ref_area11/1 -> Switch2/1
  [tank3_empty] -> Switch2/2
  Ref_area9/1 -> Switch1/1
  [tank2_empty] -> Switch1/2
  Ref_area10/1 -> Switch/1
  [tank1_empty] -> Switch/2
  Ref_area15/1 -> Product7/2
  Product7/1 -> Switch/3
  Ref_area16/1 -> Product9/2
  Ref_area17/1 -> Product10/2
  Product10/1 -> Switch2/3
  Product9/1 -> Switch1/3
  Ref_area18/1 -> Product11/2
  Product11/1 -> Switch3/3
  Add1/1 -> Product11/1, Product10/1, Product9/1, Product7/1
  Add5/1 -> Product11/3, Product9/3, Product7/3, Product10/3
  Switch/1 -> gn2_used_tank1/1
  Switch1/1 -> gn2_used_tank2/1
  Switch2/1 -> gn2_used_tank3/1
  Switch3/1 -> gn2_used_tank4/1
